simulink model "A2_8psk_simulink"  (R2019b)
settings: Solver=VariableStepAuto  StartTime=0.0  StopTime=10  RelTol=1e-3
libraries: simulink x11, commutil2 x5, dspsrcs4 x4, commchan3 x2, commfilt2 x2, dspsigops x2, commsink2 x1, commrandsrc3 x1
settings Model: Creator=linesLK  LastModifiedBy=linesLK

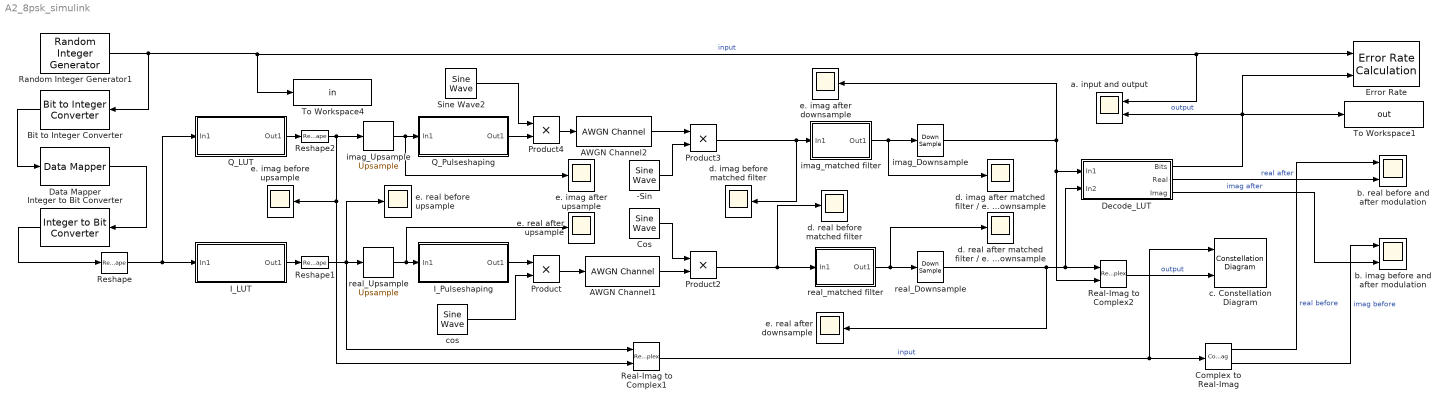
== system A2_8psk_simulink ==
  -Sin : dspsrcs4/Sine Wave  Amplitude=-1  Frequency=5  Phase=0  SampleMode=Discrete  OutComplex=Real  CompMethod=Trigonometric fcn  TableSize=Speed  SampleTime=1/80  SamplesPerFrame=8000  ResetState=Restart at time zero  OutputFrames=off  dataType=double  wordLen=16  udDataType=sfix(16)  fracBitsMode=Best precision  numFracBits=15  OutDataTypeStr=double  LastOutDataTypeStr=double
  AWGN Channel1 : commchan3/AWGN Channel  InputProcessing=Columns as channels (frame based)  seed=67  noiseMode="Signal to noise ratio  (SNR)"  EbNodB=20  EsNodB=20  SNRdB=5  bitsPerSym=3  Ps=1  Tsym=1  variance=1
      settings: SourceProductName=Communications Toolbox
  AWGN Channel2 : commchan3/AWGN Channel  InputProcessing=Columns as channels (frame based)  seed=67  noiseMode="Signal to noise ratio  (SNR)"  EbNodB=20  EsNodB=20  SNRdB=5  bitsPerSym=3  Ps=1  Tsym=1  variance=1
      settings: SourceProductName=Communications Toolbox
  Bit to Integer Converter : commutil2/Bit to Integer Converter  nbits=3  bitOrder=MSB first  signedOutputValues=Unsigned  outDtype=Inherit via internal rule  outDtypeSigned=Inherit via internal rule
      settings: SourceProductName=Communications Toolbox
  Complex to Real-Imag : ComplexToRealImag
  Cos : dspsrcs4/Sine Wave  Amplitude=1  Frequency=5  Phase=pi/2  SampleMode=Discrete  OutComplex=Real  CompMethod=Trigonometric fcn  TableSize=Speed  SampleTime=1/80  SamplesPerFrame=8000  ResetState=Restart at time zero  OutputFrames=off  dataType=double  wordLen=16  udDataType=sfix(16)  fracBitsMode=Best precision  numFracBits=15  OutDataTypeStr=double  LastOutDataTypeStr=double
  Data Mapper : commutil2/Data Mapper  MapMode=Binary to Gray  M=8  MapVec=[0 1 3 2 7 6 4 5]
      settings: SourceProductName=Communications Toolbox  SourceProductBaseCode=CM
  Decode_LUT : Subsystem
  Error Rate : commsink2/Error Rate Calculation  N=0  st_delay=0  cp_mode=Entire frame  subframe=[]  PMode=Workspace  WsName=Error  RsMode2=off  stop=off  numErr=100  maxBits=1e6
      settings: SourceProductName=Communications Toolbox
  I_LUT : Subsystem
  I_Pulseshaping : Subsystem
  Integer to Bit Converter : commutil2/Integer to Bit Converter  nbits=3  signedInputValues=Unsigned  bitOrder=MSB first  outDtype=Inherit via internal rule
      settings: SourceProductName=Communications Toolbox
  Product{,2..4} (4 alike) : Product
  Q_LUT : Subsystem
  Q_Pulseshaping : Subsystem
  Random Integer Generator1 : commrandsrc3/Random Integer Generator  SetSize=2  SeedSource=Auto  Seed=0  SampleTime=1  SamplesPerFrame=300  OutputDataType=double  SimulateUsing=Interpreted execution
      settings: SourceProductName=Communications Toolbox
  Real-Imag to Complex1 : RealImagToComplex
  Real-Imag to Complex2 : RealImagToComplex
  Reshape : Reshape  OutputDimensionality=Customize  OutputDimensions=[3,100]
  Reshape1 : Reshape  OutputDimensionality=Customize  OutputDimensions=[100,1]
  Reshape2 : Reshape  OutputDimensionality=Customize  OutputDimensions=[100,1]
  Sine Wave2 : dspsrcs4/Sine Wave  Amplitude=-1  Frequency=5  Phase=0  SampleMode=Discrete  OutComplex=Real  CompMethod=Trigonometric fcn  TableSize=Speed  SampleTime=1/80  SamplesPerFrame=8000  ResetState=Restart at time zero  OutputFrames=off  dataType=double  wordLen=16  udDataType=sfix(16)  fracBitsMode=Best precision  numFracBits=15  OutDataTypeStr=double  LastOutDataTypeStr=double
  To Workspace1 : ToWorkspace  VariableName=out  SampleTime=-1
  To Workspace4 : ToWorkspace  VariableName=in  SampleTime=-1
      settings: Save2DSignal=2-D array (concatenate along first dimension)
  a. input and output : Scope  NumInputPorts=2
  b. imag before and after modulation : Scope  NumInputPorts=2
  b. real before and after modulation : Scope  NumInputPorts=2
  c. Constellation Diagram : ConstellationDiagram  NumInputPorts=2
  cos : dspsrcs4/Sine Wave  Amplitude=1  Frequency=5  Phase=pi/2  SampleMode=Discrete  OutComplex=Real  CompMethod=Trigonometric fcn  TableSize=Speed  SampleTime=1/80  SamplesPerFrame=8000  ResetState=Restart at time zero  OutputFrames=off  dataType=double  wordLen=16  udDataType=sfix(16)  fracBitsMode=Best precision  numFracBits=15  OutDataTypeStr=double  LastOutDataTypeStr=double
  d. imag after matched filter / e. before downsample : Scope
  d. imag before matched filter : Scope
  d. real after matched filter / e. before downsample : Scope
  d. real before matched filter : Scope
  e. imag after downsample : Scope
  e. imag after upsample : Scope
  e. imag before upsample : Scope
  e. real after downsample : Scope
  e. real after upsample : Scope
  e. real before upsample : Scope
  imag_Downsample : DownSample  N=80  phase=79
  imag_Upsample : dspsigops/Upsample  N=80  phase=0  InputProcessing=Columns as channels (frame based)  RateOptions=Enforce single-rate processing  ic=0  mode=Unused parameter value
  imag_matched filter : Subsystem
  real_Downsample : DownSample  N=80  phase=79
  "real_Upsample " : dspsigops/Upsample  N=80  phase=0  InputProcessing=Columns as channels (frame based)  RateOptions=Enforce single-rate processing  ic=0  mode=Unused parameter value
  real_matched filter : Subsystem
  wires:
  Random Integer Generator1/1 -> Bit to Integer Converter/1, To Workspace4/1, a. input and output/1, Error Rate/1  "input"
  I_LUT/1(Out1) -> Reshape1/1
  Product/1 -> AWGN Channel1/1
  Real-Imag to Complex1/1 -> Complex to Real-Imag/1, c. Constellation Diagram/1  "input"
  imag_Upsample/1 -> Q_Pulseshaping/1(In1), e. imag after upsample/1
  Decode_LUT/1(Bits) -> To Workspace1/1, Error Rate/2, a. input and output/2  "output"
  "real_Upsample "/1 -> e. real after upsample/1, I_Pulseshaping/1(In1)
  real_matched filter/1(Out1) -> real_Downsample/1, d. real after matched filter / e. before downsample/1
  Q_LUT/1(Out1) -> Reshape2/1
  I_Pulseshaping/1(Out1) -> Product/1
  Cos/1 -> Product2/1
  imag_matched filter/1(Out1) -> imag_Downsample/1, d. imag after matched filter / e. before downsample/1
  Decode_LUT/3(Imag) -> b. imag before and after modulation/2  "imag after"
  AWGN Channel1/1 -> Product2/2
  Real-Imag to Complex2/1 -> c. Constellation Diagram/2  "output"
  cos/1 -> Product/2
  -Sin/1 -> Product3/2
  Reshape/1 -> Q_LUT/1(In1), I_LUT/1(In1)
  imag_Downsample/1 -> Real-Imag to Complex2/2, Decode_LUT/1(In1), e. imag after downsample/1
  real_Downsample/1 -> Decode_LUT/2(In2), Real-Imag to Complex2/1, e. real after downsample/1
  Product2/1 -> real_matched filter/1(In1), d. real before matched filter/1
  Reshape2/1 -> imag_Upsample/1, e. imag before upsample/1, Real-Imag to Complex1/2
  Reshape1/1 -> e. real before upsample/1, "real_Upsample "/1, Real-Imag to Complex1/1
  Decode_LUT/2(Real) -> b. real before and after modulation/2  "real after"
  Complex to Real-Imag/1 -> b. real before and after modulation/1  "real before"
  Complex to Real-Imag/2 -> b. imag before and after modulation/1  "imag before"
  Product3/1 -> imag_matched filter/1(In1), d. imag before matched filter/1
  Q_Pulseshaping/1(Out1) -> Product4/2
  Product4/1 -> AWGN Channel2/1
  AWGN Channel2/1 -> Product3/1
  Sine Wave2/1 -> Product4/1
  Bit to Integer Converter/1 -> Data Mapper/1
  Data Mapper/1 -> Integer to Bit Converter/1
  Integer to Bit Converter/1 -> Reshape/1

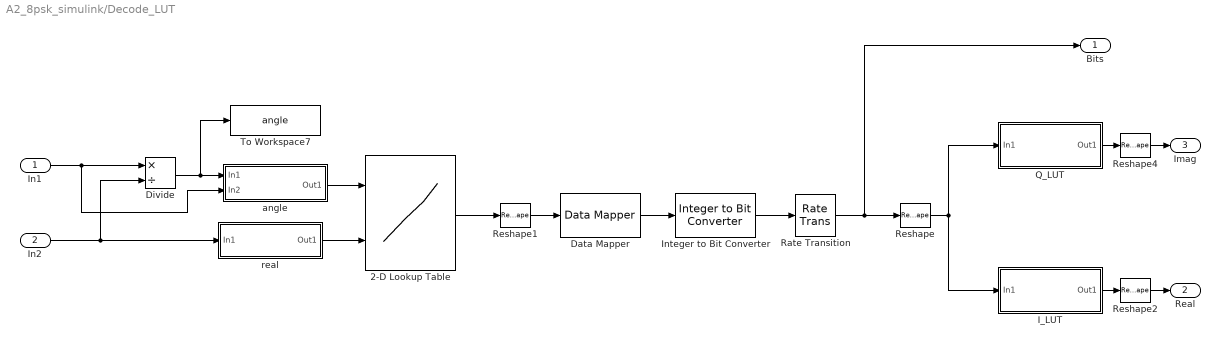
== system A2_8psk_simulink/Decode_LUT ==
  In1 : Inport
  In2 : Inport  Port=2
  2-D Lookup Table : Lookup_n-D  BreakpointsForDimension1=[-2,-1,0,1,2]  BreakpointsForDimension2=[-1,1]  Table=reshape([5,2,6,7,3,5,4,0,1,3],5,2)  InternalRulePriority=Speed  RndMeth=Simplest  InputSameDT=on
  Data Mapper : commutil2/Data Mapper  MapMode=Gray to Binary  M=8  MapVec=[0 1 3 2 7 6 4 5]
      settings: SourceProductName=Communications Toolbox  SourceProductBaseCode=CM
  Divide : Product  Inputs=*/
  I_LUT : Subsystem
  Integer to Bit Converter : commutil2/Integer to Bit Converter  nbits=3  signedInputValues=Unsigned  bitOrder=MSB first  outDtype=Inherit via internal rule
      settings: SourceProductName=Communications Toolbox
  Q_LUT : Subsystem
  Rate Transition : RateTransition  OutPortSampleTime=300
  Reshape : Reshape  OutputDimensionality=Customize  OutputDimensions=[3,100]
  Reshape1 : Reshape  OutputDimensionality=Customize  OutputDimensions=[100,1]
  Reshape2 : Reshape  OutputDimensionality=Customize  OutputDimensions=[100,1]
  Reshape4 : Reshape  OutputDimensionality=Customize  OutputDimensions=[100,1]
  To Workspace7 : ToWorkspace  VariableName=angle  SampleTime=-1
      settings: Save2DSignal=2-D array (concatenate along first dimension)
  angle : Subsystem
  real : Subsystem
  Bits : Outport
  Real : Outport  Port=2
  Imag : Outport  Port=3
  wires:
  In1/1 -> angle/2(In2), Divide/1
  In2/1 -> Divide/2, real/1(In1)
  Divide/1 -> To Workspace7/1, angle/1(In1)
  angle/1(Out1) -> 2-D Lookup Table/1
  real/1(Out1) -> 2-D Lookup Table/2
  Q_LUT/1(Out1) -> Reshape4/1
  Reshape/1 -> Q_LUT/1(In1), I_LUT/1(In1)
  I_LUT/1(Out1) -> Reshape2/1
  2-D Lookup Table/1 -> Reshape1/1
  Rate Transition/1 -> Reshape/1, Bits/1
  Reshape4/1 -> Imag/1
  Reshape2/1 -> Real/1
  Reshape1/1 -> Data Mapper/1
  Data Mapper/1 -> Integer to Bit Converter/1
  Integer to Bit Converter/1 -> Rate Transition/1

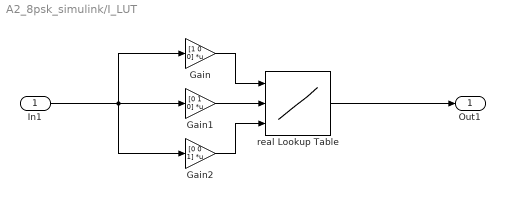
== system A2_8psk_simulink/I_LUT ==
  In1 : Inport
  Gain : Gain  Gain=[1 0 0]  Multiplication=Matrix(K*u)
  Gain1 : Gain  Gain=[0 1 0]  Multiplication=Matrix(K*u)
  Gain2 : Gain  Gain=[0 0 1]  Multiplication=Matrix(K*u)
  real Lookup Table : Lookup_n-D  NumberOfTableDimensions=3  BreakpointsForDimension1=[0,1]  BreakpointsForDimension2=[0,1]  BreakpointsForDimension3=[0,1]  Table=reshape([1,sqrt(2)/2,-sqrt(2)/2,-1,sqrt(2)/2,0,0,-sqrt(2)/2],2,2,2)  InternalRulePriority=Speed  RndMeth=Simplest  InputSameDT=on
  Out1 : Outport
  wires:
  Gain2/1 -> real Lookup Table/3
  In1/1 -> Gain/1, Gain1/1, Gain2/1
  Gain/1 -> real Lookup Table/1
  Gain1/1 -> real Lookup Table/2
  real Lookup Table/1 -> Out1/1

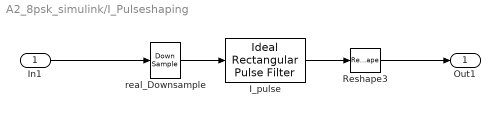
== system A2_8psk_simulink/I_Pulseshaping ==
  In1 : Inport
  I_pulse : commfilt2/Ideal Rectangular Pulse Filter  pulseLen=80  pulseDelay=0  InputProcessing=Columns as channels (frame based)  RateOptions=Enforce single-rate processing  sampMode=Mute  normCheck=off  normMode=Sum of samples  filterGain=1  saveAsFlag=0  roundingMode=Floor  overflowMode=off  firstCoeffDataTypeStr=Inherit: Same word length as input  firstCoeffMin=[]  firstCoeffMax=[]  firstCoeffLastDataTypeStr=Inherit: Same word length as input  outputDataTypeStr=Inherit: Same as accumulator  outputMin=[]  outputMax=[]  outputLastDataTypeStr=Inherit: Same as accumulator
      settings: SourceProductName=Communications Toolbox  SourceProductBaseCode=CM
  Reshape3 : Reshape  OutputDimensionality=Customize  OutputDimensions=[8000,1]
  real_Downsample : DownSample  N=80
  Out1 : Outport
  wires:
  Reshape3/1 -> Out1/1
  real_Downsample/1 -> I_pulse/1
  In1/1 -> real_Downsample/1
  I_pulse/1 -> Reshape3/1

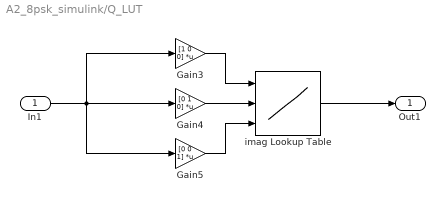
== system A2_8psk_simulink/Q_LUT ==
  In1 : Inport
  Gain3 : Gain  Gain=[1 0 0]  Multiplication=Matrix(K*u)
  Gain4 : Gain  Gain=[0 1 0]  Multiplication=Matrix(K*u)
  Gain5 : Gain  Gain=[0 0 1]  Multiplication=Matrix(K*u)
  imag Lookup Table : Lookup_n-D  NumberOfTableDimensions=3  BreakpointsForDimension1=[0,1]  BreakpointsForDimension2=[0,1]  BreakpointsForDimension3=[0,1]  Table=reshape([0,-sqrt(2)/2,sqrt(2)/2,0,sqrt(2)/2,-1,1,-sqrt(2)/2],2,2,2)  InternalRulePriority=Speed  RndMeth=Simplest  InputSameDT=on
  Out1 : Outport
  wires:
  imag Lookup Table/1 -> Out1/1
  Gain3/1 -> imag Lookup Table/1
  Gain5/1 -> imag Lookup Table/3
  Gain4/1 -> imag Lookup Table/2
  In1/1 -> Gain5/1, Gain4/1, Gain3/1

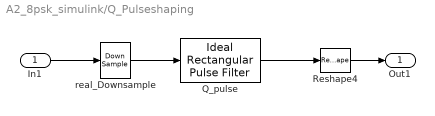
== system A2_8psk_simulink/Q_Pulseshaping ==
  In1 : Inport
  Q_pulse : commfilt2/Ideal Rectangular Pulse Filter  pulseLen=80  pulseDelay=0  InputProcessing=Columns as channels (frame based)  RateOptions=Enforce single-rate processing  sampMode=Mute  normCheck=off  normMode=Sum of samples  filterGain=1  saveAsFlag=0  roundingMode=Floor  overflowMode=off  firstCoeffDataTypeStr=Inherit: Same word length as input  firstCoeffMin=[]  firstCoeffMax=[]  firstCoeffLastDataTypeStr=Inherit: Same word length as input  outputDataTypeStr=Inherit: Same as accumulator  outputMin=[]  outputMax=[]  outputLastDataTypeStr=Inherit: Same as accumulator
      settings: SourceProductName=Communications Toolbox  SourceProductBaseCode=CM
  Reshape4 : Reshape  OutputDimensionality=Customize  OutputDimensions=[8000,1]
  real_Downsample : DownSample  N=80
  Out1 : Outport
  wires:
  real_Downsample/1 -> Q_pulse/1
  Q_pulse/1 -> Reshape4/1
  Reshape4/1 -> Out1/1
  In1/1 -> real_Downsample/1

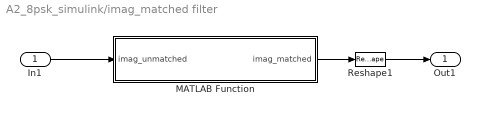
== system A2_8psk_simulink/imag_matched filter ==
  In1 : Inport
  MATLAB Function : MATLAB Function  TreatAsAtomicUnit=on
  Reshape1 : Reshape  OutputDimensionality=Customize  OutputDimensions=[8000,1]
  Out1 : Outport
  wires:
  MATLAB Function/1(imag_matched) -> Reshape1/1
  In1/1 -> MATLAB Function/1(imag_unmatched)
  Reshape1/1 -> Out1/1

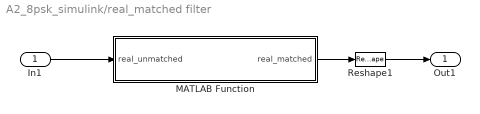
== system A2_8psk_simulink/real_matched filter ==
  In1 : Inport
  MATLAB Function : MATLAB Function  TreatAsAtomicUnit=on
  Reshape1 : Reshape  OutputDimensionality=Customize  OutputDimensions=[8000,1]
  Out1 : Outport
  wires:
  MATLAB Function/1(real_matched) -> Reshape1/1
  In1/1 -> MATLAB Function/1(real_unmatched)
  Reshape1/1 -> Out1/1

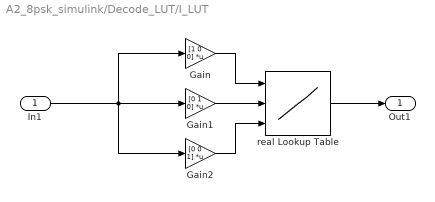
== system A2_8psk_simulink/Decode_LUT/I_LUT ==
  In1 : Inport
  Gain : Gain  Gain=[1 0 0]  Multiplication=Matrix(K*u)
  Gain1 : Gain  Gain=[0 1 0]  Multiplication=Matrix(K*u)
  Gain2 : Gain  Gain=[0 0 1]  Multiplication=Matrix(K*u)
  real Lookup Table : Lookup_n-D  NumberOfTableDimensions=3  BreakpointsForDimension1=[0,1]  BreakpointsForDimension2=[0,1]  BreakpointsForDimension3=[0,1]  Table=reshape([1,sqrt(2)/2,-sqrt(2)/2,-1,sqrt(2)/2,0,0,-sqrt(2)/2],2,2,2)  InternalRulePriority=Speed  RndMeth=Simplest  InputSameDT=on
  Out1 : Outport
  wires:
  Gain2/1 -> real Lookup Table/3
  In1/1 -> Gain/1, Gain1/1, Gain2/1
  Gain/1 -> real Lookup Table/1
  Gain1/1 -> real Lookup Table/2
  real Lookup Table/1 -> Out1/1

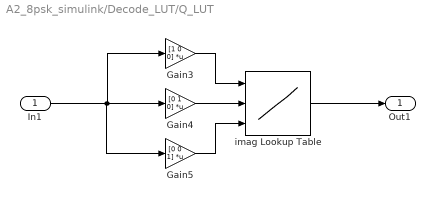
== system A2_8psk_simulink/Decode_LUT/Q_LUT ==
  In1 : Inport
  Gain3 : Gain  Gain=[1 0 0]  Multiplication=Matrix(K*u)
  Gain4 : Gain  Gain=[0 1 0]  Multiplication=Matrix(K*u)
  Gain5 : Gain  Gain=[0 0 1]  Multiplication=Matrix(K*u)
  imag Lookup Table : Lookup_n-D  NumberOfTableDimensions=3  BreakpointsForDimension1=[0,1]  BreakpointsForDimension2=[0,1]  BreakpointsForDimension3=[0,1]  Table=reshape([0,-sqrt(2)/2,sqrt(2)/2,0,sqrt(2)/2,-1,1,-sqrt(2)/2],2,2,2)  InternalRulePriority=Speed  RndMeth=Simplest  InputSameDT=on
  Out1 : Outport
  wires:
  imag Lookup Table/1 -> Out1/1
  Gain3/1 -> imag Lookup Table/1
  Gain5/1 -> imag Lookup Table/3
  Gain4/1 -> imag Lookup Table/2
  In1/1 -> Gain5/1, Gain3/1, Gain4/1

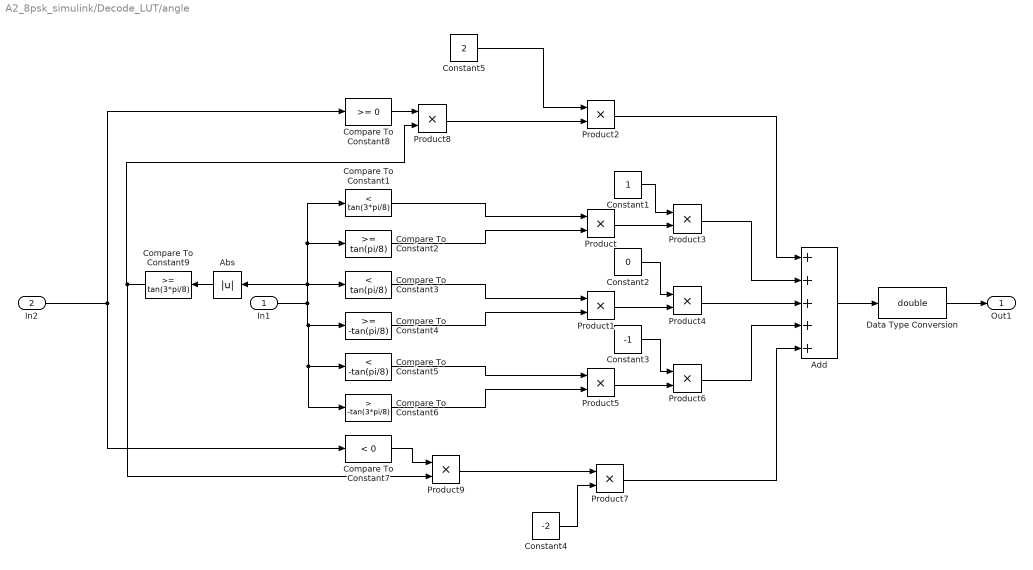
== system A2_8psk_simulink/Decode_LUT/angle ==
  In1 : Inport
  In2 : Inport  Port=2
  Abs : Abs
  Add : Sum  Inputs=+++++
  Compare To Constant1 : simulink/Logic and Bit Operations/Compare To Constant  relop=<  const=tan(3*pi/8)  OutDataTypeStr=boolean
  Compare To Constant2 : simulink/Logic and Bit Operations/Compare To Constant  relop=>=  const=tan(pi/8)  OutDataTypeStr=boolean
  Compare To Constant3 : simulink/Logic and Bit Operations/Compare To Constant  relop=<  const=tan(pi/8)  OutDataTypeStr=boolean
  Compare To Constant4 : simulink/Logic and Bit Operations/Compare To Constant  relop=>=  const=-tan(pi/8)  OutDataTypeStr=boolean
  Compare To Constant5 : simulink/Logic and Bit Operations/Compare To Constant  relop=<  const=-tan(pi/8)  OutDataTypeStr=boolean
  Compare To Constant6 : simulink/Logic and Bit Operations/Compare To Constant  relop=>  const=-tan(3*pi/8)  OutDataTypeStr=boolean
  Compare To Constant7 : simulink/Logic and Bit Operations/Compare To Constant  relop=<  const=0  OutDataTypeStr=boolean
  Compare To Constant8 : simulink/Logic and Bit Operations/Compare To Constant  relop=>=  const=0  OutDataTypeStr=boolean
  Compare To Constant9 : simulink/Logic and Bit Operations/Compare To Constant  relop=>=  const=tan(3*pi/8)  OutDataTypeStr=boolean
  Constant1 : Constant
  Constant2 : Constant  Value=0
  Constant3 : Constant  Value=-1
  Constant4 : Constant  Value=-2
  Constant5 : Constant  Value=2
  Data Type Conversion : DataTypeConversion  OutDataTypeStr=double
  Product{,1..9} (10 alike) : Product
  Out1 : Outport
  wires:
  In1/1 -> Compare To Constant2/1, Compare To Constant1/1, Abs/1, Compare To Constant3/1, Compare To Constant5/1, Compare To Constant6/1, Compare To Constant4/1
  Compare To Constant1/1 -> Product/1
  Compare To Constant2/1 -> Product/2
  Compare To Constant3/1 -> Product1/1
  Compare To Constant4/1 -> Product1/2
  Constant1/1 -> Product3/1
  Product/1 -> Product3/2
  Product1/1 -> Product4/2
  Constant2/1 -> Product4/1
  Compare To Constant6/1 -> Product5/2
  Compare To Constant5/1 -> Product5/1
  Constant3/1 -> Product6/1
  Product5/1 -> Product6/2
  Constant4/1 -> Product7/2
  Product4/1 -> Add/3
  Product3/1 -> Add/2
  Product6/1 -> Add/4
  Product7/1 -> Add/5
  Add/1 -> Data Type Conversion/1
  Data Type Conversion/1 -> Out1/1
  In2/1 -> Compare To Constant7/1, Compare To Constant8/1
  Constant5/1 -> Product2/1
  Product2/1 -> Add/1
  Abs/1 -> Compare To Constant9/1
  Compare To Constant9/1 -> Product9/2, Product8/2
  Compare To Constant8/1 -> Product8/1
  Product8/1 -> Product2/2
  Compare To Constant7/1 -> Product9/1
  Product9/1 -> Product7/1

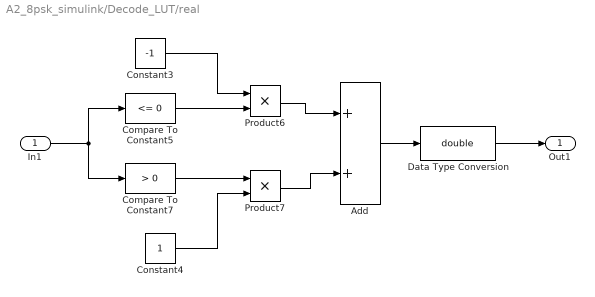
== system A2_8psk_simulink/Decode_LUT/real ==
  In1 : Inport
  Add : Sum
  Compare To Constant5 : simulink/Logic and Bit Operations/Compare To Constant  relop=<=  const=0  OutDataTypeStr=boolean
  Compare To Constant7 : simulink/Logic and Bit Operations/Compare To Constant  relop=>  const=0  OutDataTypeStr=boolean
  Constant3 : Constant  Value=-1
  Constant4 : Constant
  Data Type Conversion : DataTypeConversion  OutDataTypeStr=double
  Product6 : Product
  Product7 : Product
  Out1 : Outport
  wires:
  Constant3/1 -> Product6/1
  Compare To Constant5/1 -> Product6/2
  Compare To Constant7/1 -> Product7/1
  Constant4/1 -> Product7/2
  Add/1 -> Data Type Conversion/1
  Data Type Conversion/1 -> Out1/1
  In1/1 -> Compare To Constant7/1, Compare To Constant5/1
  Product6/1 -> Add/1
  Product7/1 -> Add/2

== matlab function A2_8psk_simulink/real_matched filter/MATLAB Function ==
  data: real_unmatched input; real_matched output
function real_matched = fcn(real_unmatched)
F = ones(1,80);
real_matched = filter(F,1,real_unmatched)/40;

== matlab function A2_8psk_simulink/imag_matched filter/MATLAB Function ==
  data: imag_unmatched input; imag_matched output
function imag_matched = fcn(imag_unmatched)
F = ones(1,80);
imag_matched = filter(F,1,imag_unmatched)/40;
